simulink model "EPT"  (R2019b)
settings: Solver=FixedStepDiscrete  StartTime=0.0  StopTime=5  FixedStep=0.005  RelTol=1e-3  EnableMultiTasking=on
PreLoadFcn:
  | try, model_open; catch, disp('Error occurred while executing model pre-load callback: model_open.m'); disp('Please assure that the MATLAB working directory is set to the model directory before opening.'); end
InitFcn:
  | try, model_open; catch, end
undefined symbols (not defined in the file or in its folder): Bridge, GCM, H, ln, raptor_get_param_eval, raptor_get_safe_string, raptor_xcp_function
libraries: Raptor_lib x2810, simulink x374, hdlsllib x19
(part 17 of 45)

== system EPT/Foreground_TimeBase_5ms/CAN/CAN2_exec/Remote DA /Remote DA Status G23 (CHGer) ==
  Trigger : TriggerPort  VariantControl=Variant  PortDimensions=1
  raptor_can_txmsg : Raptor_lib/CAN/raptor_can_txmsg  canDefinition=struct('dbcFile', 'EPTvsRemoteDA.dbc','message', 'Remote_DA_Status_G23','comment', '','signals', {{'EPT_OBC_STOP_CTRL','EPT_OBC_IOUT_CMD','EPT_OBC_VOUT_CMD','EPT_OBC_STA','EPT_OBC_CURR','EPT_OBC_VOLT','EPT_OBC_TEMP','EPT_OBC_EW_CODE'}},'enabled', [ 1 1 1 1 1 1 1 1;],'canBus', '''CAN2''','messageID', [ 405008116;],'idMask', [ 536870911;],'payloadMask', [],'payloadValue', [],'period', [ 0;],'mailbox', '','queueSize', [ 1;],'label', [ 1;],'ver', [ 2;],'showID', [ 0;],'showRaw', [ 0;],'fill', [ 0;],'editID', [ 0;],'signalOrder', [ 2;])  canBus='CAN2'  queueSize=1  payloadMask=[]  payloadValue=[]  period=0  showID=0  label=1  idMask=hex2dec('1FFFFFFF')  fill=0  id=405008116  showRaw=0  signalOrder=2  signalInfo={{struct('Name', 'EPT_OBC_VOUT_CMD','Startbit', [ 0;],'SignalSize', [ 8;],'ByteOrder', 'LittleEndian','ValueType', 'UNSIGNED','Class', 'uint8','Signed', [ 0;],'Factor', [ 0.4;],'Offset', [ 0;],'Min', [ 0;],'Max', [ 100;],'Units', '%(Max_Vbatt)','Comment', '','StartBit', [ 16;]),struct('Name', 'EPT_OBC_VOLT','Startbit', [ 0;],'SignalSize', [ 8;],'ByteOrder', 'LittleEndian','ValueType', 'UNSIGNED','Class', 'uint8','Signed', [ 0;],'Factor', [ 0.4;],'Offset', [ 0;],'Min', [ 0;],'Max', [ 100;],'Units', '%(Max_Vchger)','Comment', '','StartBit', [ 40;]),struct('Name', 'EPT_OBC_TEMP','Startbit', [ 0;],'SignalSize', [ 8;],'ByteOrder', 'LittleEndian','ValueType', 'UNSIGNED','Class', 'uint8','Signed', [ 0;],'Factor', [ 1;],'Offset', [ -40;],'Min', [ -40;],'Max', [ 210;],'Units', 'degC','Comment', '','StartBit', [ 48;]),struct('Name', 'EPT_OBC_STOP_CTRL','Startbit', [ 0;],'SignalSize', [ 1;],'ByteOrder', 'LittleEndian','ValueType', 'UNSIGNED','Class', 'uint8','Signed', [ 0;],'Factor', [ 1;],'Offset', [ 0;],'Min', [ 0;],'Max', [ 0;],'Units', '','Comment', '','StartBit', [ 0;]),struct('Name', 'EPT_OBC_STA','Startbit', [ 0;],'SignalSize', [ 1;],'ByteOrder', 'LittleEndian','ValueType', 'UNSIGNED','Class', 'uint8','Signed', [ 0;],'Factor', [ 1;],'Offset', [ 0;],'Min', [ 0;],'Max', [ 0;],'Units', '','Comment', '','StartBit', [ 24;]),struct('Name', 'EPT_OBC_IOUT_CMD','Startbit', [ 0;],'SignalSize', [ 8;],'ByteOrder', 'LittleEndian','ValueType', 'UNSIGNED','Class', 'uint8','Signed', [ 0;],'Factor', [ 0.4;],'Offset', [ 0;],'Min', [ 0;],'Max', [ 100;],'Units', '%(Max Ichger)','Comment', '','StartBit', [ 8;]),struct('Name', 'EPT_OBC_EW_CODE','Startbit', [ 0;],'SignalSize', [ 8;],'ByteOrder', 'LittleEndian','ValueType', 'UNSIGNED','Class', 'uint8','Signed', [ 0;],'Factor', [ 1;],'Offset', [ 0;],'Min', [ 0;],'Max', [ 0;],'Units', '','Comment', '','StartBit', [ 56;]),struct('Name', 'EPT_OBC_CURR','Startbit', [ 0;],'SignalSize', [ 8;],'ByteOrder', 'LittleEndian','ValueType', 'UNSIGNED','Class', 'uint8','Signed', [ 0;],'Factor', [ 0.4;],'Offset', [ 0;],'Min', [ 0;],'Max', [ 100;],'Units', '%(Max Ichger)','Comment', '','StartBit', [ 32;])}}
      settings: SourceProductName=Raptor
  raptor_data_read1 : Raptor_lib/Data Storage/raptor_data_read  dataName='EPT_OBC_VOUT_CMD'  dataShape=Scalar  idxSource=Input  idxRow=1  idxCol=1
      settings: SourceProductName=Raptor
  raptor_data_read2 : Raptor_lib/Data Storage/raptor_data_read  dataName='Read_OBC_Temp'  dataShape=Scalar  idxSource=Input  idxRow=1  idxCol=1
      settings: SourceProductName=Raptor
  raptor_data_read3 : Raptor_lib/Data Storage/raptor_data_read  dataName='EPT_OBC_EN'  dataShape=Scalar  idxSource=Input  idxRow=1  idxCol=1
      settings: SourceProductName=Raptor
  raptor_data_read4 : Raptor_lib/Data Storage/raptor_data_read  dataName='EPT_OBC_STA'  dataShape=Scalar  idxSource=Input  idxRow=1  idxCol=1
      settings: SourceProductName=Raptor
  raptor_data_read5 : Raptor_lib/Data Storage/raptor_data_read  dataName='Read_OBC_Vout'  dataShape=Scalar  idxSource=Input  idxRow=1  idxCol=1
      settings: SourceProductName=Raptor
  raptor_data_read6 : Raptor_lib/Data Storage/raptor_data_read  dataName='Read_OBC_Cout'  dataShape=Scalar  idxSource=Input  idxRow=1  idxCol=1
      settings: SourceProductName=Raptor
  raptor_data_read7 : Raptor_lib/Data Storage/raptor_data_read  dataName='EPT_OBC_IOUT_CMD'  dataShape=Scalar  idxSource=Input  idxRow=1  idxCol=1
      settings: SourceProductName=Raptor
  raptor_data_read8 : Raptor_lib/Data Storage/raptor_data_read  dataName='Read_OBC_Status'  dataShape=Scalar  idxSource=Input  idxRow=1  idxCol=1
      settings: SourceProductName=Raptor
  wires:
  raptor_data_read1/1 -> raptor_can_txmsg/3  "EPT_OBC_VOUT_CMD"
  raptor_data_read3/1 -> raptor_can_txmsg/1  "EPT_OBC_STOP_CTRL"
  raptor_data_read4/1 -> raptor_can_txmsg/4  "EPT_OBC_STA"
  raptor_data_read2/1 -> raptor_can_txmsg/7  "EPT_OBC_TEMP"
  raptor_data_read5/1 -> raptor_can_txmsg/6  "EPT_OBC_VOLT"
  raptor_data_read6/1 -> raptor_can_txmsg/5  "EPT_OBC_CURR"
  raptor_data_read7/1 -> raptor_can_txmsg/2  "EPT_OBC_IOUT_CMD"
  raptor_data_read8/1 -> raptor_can_txmsg/8  "EPT_OBC_EW_CODE"

== system EPT/Foreground_TimeBase_5ms/CAN/CAN2_exec/Remote DA /Remote DA Status G30 (ESS-SWCU) ==
  Trigger : TriggerPort  VariantControl=Variant  PortDimensions=1
  raptor_can_txmsg : Raptor_lib/CAN/raptor_can_txmsg  canDefinition=struct('dbcFile', 'EPTvsRemoteDA.dbc','message', 'Remote_DA_Status_G30','comment', '','signals', {{'EPT_SWCU_READY','EPT_BPSWU_READY','EPT_PWCU_READY','EPT_SWCU_HV_ENABLED','EPT_SWAP_REQ','EPT_BPSWU_INSTALL_NUM','EPT_SWCU_EW_CODE','EPT_BPSWU_FCCAP','EPT_BPSWU_RSOC','EPT_BPSWU_TEMP','EPT_PWCU_CURR_MAX','EPT_PWCU_CURR','EPT_PWCU_TEMP'}},'enabled', [ 1 1 1 1 1 1 1 1 1 1 1 1 1;],'canBus', '''CAN2''','messageID', [ 405860084;],'idMask', [ 536870911;],'payloadMask', [],'payloadValue', [],'period', [ 0;],'mailbox', '','queueSize', [ 1;],'label', [ 0;],'ver', [ 2;],'showID', [ 0;],'showRaw', [ 0;],'fill', [ 0;],'editID', [ 0;],'signalOrder', [ 2;])  canBus='CAN2'  queueSize=1  payloadMask=[]  payloadValue=[]  period=0  showID=0  label=0  idMask=hex2dec('1FFFFFFF')  fill=0  id=405860084  showRaw=0  signalOrder=2  signalInfo={{struct('Name', 'EPT_BPSWU_TEMP','Startbit', [ 0;],'SignalSize', [ 8;],'ByteOrder', 'LittleEndian','ValueType', 'UNSIGNED','Class', 'uint8','Signed', [ 0;],'Factor', [ 1;],'Offset', [ -40;],'Min', [ -40;],'Max', [ 210;],'Units', 'degC','Comment', '','StartBit', [ 32;]),struct('Name', 'EPT_BPSWU_RSOC','Startbit', [ 0;],'SignalSize', [ 8;],'ByteOrder', 'LittleEndian','ValueType', 'UNSIGNED','Class', 'uint8','Signed', [ 0;],'Factor', [ 0.5;],'Offset', [ -12.5;],'Min', [ -12.5;],'Max', [ 112.5;],'Units', 'pct','Comment', '','StartBit', [ 24;]),struct('Name', 'EPT_BPSWU_FCCAP','Startbit', [ 0;],'SignalSize', [ 8;],'ByteOrder', 'LittleEndian','ValueType', 'UNSIGNED','Class', 'uint8','Signed', [ 0;],'Factor', [ 0.4;],'Offset', [ 0;],'Min', [ 0;],'Max', [ 100;],'Units', 'pct (Max_Ah)','Comment', '','StartBit', [ 16;]),struct('Name', 'EPT_SWCU_EW_CODE','Startbit', [ 0;],'SignalSize', [ 8;],'ByteOrder', 'LittleEndian','ValueType', 'UNSIGNED','Class', 'uint8','Signed', [ 0;],'Factor', [ 1;],'Offset', [ 0;],'Min', [ 0;],'Max', [ 0;],'Units', '','Comment', '','StartBit', [ 8;]),struct('Name', 'EPT_PWCU_TEMP','Startbit', [ 0;],'SignalSize', [ 8;],'ByteOrder', 'LittleEndian','ValueType', 'UNSIGNED','Class', 'uint8','Signed', [ 0;],'Factor', [ 1;],'Offset', [ -40;],'Min', [ -40;],'Max', [ 210;],'Units', 'degC','Comment', '','StartBit', [ 56;]),struct('Name', 'EPT_PWCU_CURR_MAX','Startbit', [ 0;],'SignalSize', [ 8;],'ByteOrder', 'LittleEndian','ValueType', 'UNSIGNED','Class', 'uint8','Signed', [ 0;],'Factor', [ 0.4;],'Offset', [ 0;],'Min', [ 0;],'Max', [ 100;],'Units', '% (Imax)','Comment', '','StartBit', [ 40;]),struct('Name', 'EPT_PWCU_CURR','Startbit', [ 0;],'SignalSize', [ 8;],'ByteOrder', 'LittleEndian','ValueType', 'UNSIGNED','Class', 'uint8','Signed', [ 0;],'Factor', [ 0.4;],'Offset', [ 0;],'Min', [ 0;],'Max', [ 100;],'Units', '% (Imax)','Comment', '','StartBit', [ 48;]),struct('Name', 'EPT_BPSWU_INSTALL_NUM','Startbit', [ 0;],'SignalSize', [ 3;],'ByteOrder', 'LittleEndian','ValueType', 'UNSIGNED','Class', 'uint8','Signed', [ 0;],'Factor', [ 1;],'Offset', [ 0;],'Min', [ 0;],'Max', [ 0;],'Units', '','Comment', '','StartBit', [ 5;]),struct('Name', 'EPT_SWCU_READY','Startbit', [ 0;],'SignalSize', [ 1;],'ByteOrder', 'LittleEndian','ValueType', 'UNSIGNED','Class', 'uint8','Signed', [ 0;],'Factor', [ 1;],'Offset', [ 0;],'Min', [ 0;],'Max', [ 0;],'Units', '','Comment', '','StartBit', [ 0;]),struct('Name', 'EPT_SWCU_HV_ENABLED','Startbit', [ 0;],'SignalSize', [ 1;],'ByteOrder', 'LittleEndian','ValueType', 'UNSIGNED','Class', 'uint8','Signed', [ 0;],'Factor', [ 1;],'Offset', [ 0;],'Min', [ 0;],'Max', [ 0;],'Units', '','Comment', '','StartBit', [ 3;]),struct('Name', 'EPT_SWAP_REQ','Startbit', [ 0;],'SignalSize', [ 1;],'ByteOrder', 'LittleEndian','ValueType', 'UNSIGNED','Class', 'uint8','Signed', [ 0;],'Factor', [ 1;],'Offset', [ 0;],'Min', [ 0;],'Max', [ 0;],'Units', '','Comment', '','StartBit', [ 4;]),struct('Name', 'EPT_PWCU_READY','Startbit', [ 0;],'SignalSize', [ 1;],'ByteOrder', 'LittleEndian','ValueType', 'UNSIGNED','Class', 'uint8','Signed', [ 0;],'Factor', [ 1;],'Offset', [ 0;],'Min', [ 0;],'Max', [ 0;],'Units', '','Comment', '','StartBit', [ 2;]),struct('Name', 'EPT_BPSWU_READY','Startbit', [ 0;],'SignalSize', [ 1;],'ByteOrder', 'LittleEndian','ValueType', 'UNSIGNED','Class', 'uint8','Signed', [ 0;],'Factor', [ 1;],'Offset', [ 0;],'Min', [ 0;],'Max', [ 0;],'Units', '','Comment', '','StartBit', [ 1;])}}
      settings: SourceProductName=Raptor
  raptor_data_read : Raptor_lib/Data Storage/raptor_data_read  dataName='SWCU_PWCU_READY'  dataShape=Scalar  idxSource=Input  idxRow=1  idxCol=1
      settings: SourceProductName=Raptor
  raptor_data_read1 : Raptor_lib/Data Storage/raptor_data_read  dataName='SWCU_HV_ENABLED'  dataShape=Scalar  idxSource=Input  idxRow=1  idxCol=1
      settings: SourceProductName=Raptor
  raptor_data_read10 : Raptor_lib/Data Storage/raptor_data_read  dataName='SWCU_BPSWU_FCCAP'  dataShape=Scalar  idxSource=Input  idxRow=1  idxCol=1
      settings: SourceProductName=Raptor
  raptor_data_read11 : Raptor_lib/Data Storage/raptor_data_read  dataName='SWCU_PWCU_IOUT'  dataShape=Scalar  idxSource=Input  idxRow=1  idxCol=1
      settings: SourceProductName=Raptor
  raptor_data_read2 : Raptor_lib/Data Storage/raptor_data_read  dataName='SWCU_SWAP_REQUEST'  dataShape=Scalar  idxSource=Input  idxRow=1  idxCol=1
      settings: SourceProductName=Raptor
  raptor_data_read3 : Raptor_lib/Data Storage/raptor_data_read  dataName='SWCU_BPSWU_INSTALL_NUM'  dataShape=Scalar  idxSource=Input  idxRow=1  idxCol=1
      settings: SourceProductName=Raptor
  raptor_data_read4 : Raptor_lib/Data Storage/raptor_data_read  dataName='SWCU_EW_CODE'  dataShape=Scalar  idxSource=Input  idxRow=1  idxCol=1
      settings: SourceProductName=Raptor
  raptor_data_read5 : Raptor_lib/Data Storage/raptor_data_read  dataName='SWCU_BPSWU_TEMP'  dataShape=Scalar  idxSource=Input  idxRow=1  idxCol=1
      settings: SourceProductName=Raptor
  raptor_data_read6 : Raptor_lib/Data Storage/raptor_data_read  dataName='SWCU_PWCU_TEMP'  dataShape=Scalar  idxSource=Input  idxRow=1  idxCol=1
      settings: SourceProductName=Raptor
  raptor_data_read7 : Raptor_lib/Data Storage/raptor_data_read  dataName='SWCU_BPSWU_READY'  dataShape=Scalar  idxSource=Input  idxRow=1  idxCol=1
      settings: SourceProductName=Raptor
  raptor_data_read8 : Raptor_lib/Data Storage/raptor_data_read  dataName='SWCU_READY'  dataShape=Scalar  idxSource=Input  idxRow=1  idxCol=1
      settings: SourceProductName=Raptor
  raptor_data_read9 : Raptor_lib/Data Storage/raptor_data_read  dataName='SWCU_BPSWU_RSOC'  dataShape=Scalar  idxSource=Input  idxRow=1  idxCol=1
      settings: SourceProductName=Raptor
  wires:
  raptor_data_read/1 -> raptor_can_txmsg/3
  raptor_data_read1/1 -> raptor_can_txmsg/4
  raptor_data_read2/1 -> raptor_can_txmsg/5
  raptor_data_read7/1 -> raptor_can_txmsg/2
  raptor_data_read8/1 -> raptor_can_txmsg/1
  raptor_data_read9/1 -> raptor_can_txmsg/9
  raptor_data_read10/1 -> raptor_can_txmsg/8
  raptor_data_read3/1 -> raptor_can_txmsg/6
  raptor_data_read4/1 -> raptor_can_txmsg/7
  raptor_data_read5/1 -> raptor_can_txmsg/10
  raptor_data_read6/1 -> raptor_can_txmsg/13
  raptor_data_read11/1 -> raptor_can_txmsg/12

== system EPT/Foreground_TimeBase_5ms/CAN/CAN2_exec/Remote DA /Remote DA Status G31 (ESS-SWUBP#1) ==
  Trigger : TriggerPort  VariantControl=Variant  PortDimensions=1
  raptor_can_txmsg : Raptor_lib/CAN/raptor_can_txmsg  canDefinition=struct('dbcFile', 'EPTvsRemoteDA.dbc','message', 'Remote_DA_Status_G31','comment', '','signals', {{'EPT_BPSWU1_READY','EPT_BPSWU1_HV_ENABLED','EPT_BPSWU1_EW','EPT_BPSWU1_EW_CODE','EPT_BPSWU1_FCCAP','EPT_BPSWU1_RSOC','EPT_BPSWU1_CURR','EPT_BPSWU1_VOLT','EPT_BPSWU1_TEMP','EPT_BPSWU1_VCELL_MAX','EPT_BPSWU1_VCELL_MIN'}},'enabled', [ 1 1 1 1 1 1 1 1 1 1 1;],'canBus', '''CAN2''','messageID', [ 405925620;],'idMask', [ 536870911;],'payloadMask', [],'payloadValue', [],'period', [ 0;],'mailbox', '','queueSize', [ 1;],'label', [ 0;],'ver', [ 2;],'showID', [ 0;],'showRaw', [ 0;],'fill', [ 0;],'editID', [ 0;],'signalOrder', [ 2;])  canBus='CAN2'  queueSize=1  payloadMask=[]  payloadValue=[]  period=0  showID=0  label=0  idMask=hex2dec('1FFFFFFF')  fill=0  id=405925620  showRaw=0  signalOrder=2  signalInfo={{struct('Name', 'EPT_BPSWU1_VOLT','Startbit', [ 0;],'SignalSize', [ 8;],'ByteOrder', 'LittleEndian','ValueType', 'UNSIGNED','Class', 'uint8','Signed', [ 0;],'Factor', [ 0.4;],'Offset', [ 0;],'Min', [ 0;],'Max', [ 100;],'Units', 'pct (Max_Vbatt)','Comment', '','StartBit', [ 32;]),struct('Name', 'EPT_BPSWU1_VCELL_MIN','Startbit', [ 0;],'SignalSize', [ 8;],'ByteOrder', 'LittleEndian','ValueType', 'UNSIGNED','Class', 'uint8','Signed', [ 0;],'Factor', [ 0.01;],'Offset', [ 2;],'Min', [ 2;],'Max', [ 4.5;],'Units', 'Volt','Comment', '','StartBit', [ 56;]),struct('Name', 'EPT_BPSWU1_VCELL_MAX','Startbit', [ 0;],'SignalSize', [ 8;],'ByteOrder', 'LittleEndian','ValueType', 'UNSIGNED','Class', 'uint8','Signed', [ 0;],'Factor', [ 0.01;],'Offset', [ 2;],'Min', [ 2;],'Max', [ 4.5;],'Units', 'Volt','Comment', '','StartBit', [ 48;]),struct('Name', 'EPT_BPSWU1_TEMP','Startbit', [ 0;],'SignalSize', [ 8;],'ByteOrder', 'LittleEndian','ValueType', 'UNSIGNED','Class', 'uint8','Signed', [ 0;],'Factor', [ 1;],'Offset', [ -40;],'Min', [ -40;],'Max', [ 210;],'Units', 'degC','Comment', '','StartBit', [ 40;]),struct('Name', 'EPT_BPSWU1_RSOC','Startbit', [ 0;],'SignalSize', [ 8;],'ByteOrder', 'LittleEndian','ValueType', 'UNSIGNED','Class', 'uint8','Signed', [ 0;],'Factor', [ 1;],'Offset', [ 0;],'Min', [ 0;],'Max', [ 0;],'Units', '','Comment', '','StartBit', [ 16;]),struct('Name', 'EPT_BPSWU1_FCCAP','Startbit', [ 0;],'SignalSize', [ 8;],'ByteOrder', 'LittleEndian','ValueType', 'UNSIGNED','Class', 'uint8','Signed', [ 0;],'Factor', [ 0.4;],'Offset', [ 0;],'Min', [ 0;],'Max', [ 100;],'Units', 'pct (Max_Ah)','Comment', '','StartBit', [ 8;]),struct('Name', 'EPT_BPSWU1_CURR','Startbit', [ 0;],'SignalSize', [ 8;],'ByteOrder', 'LittleEndian','ValueType', 'UNSIGNED','Class', 'uint8','Signed', [ 0;],'Factor', [ 0.8;],'Offset', [ -100;],'Min', [ -100;],'Max', [ 100;],'Units', 'pct (Max Ibatt)','Comment', '','StartBit', [ 24;]),struct('Name', 'EPT_BPSWU1_EW_CODE','Startbit', [ 0;],'SignalSize', [ 5;],'ByteOrder', 'LittleEndian','ValueType', 'UNSIGNED','Class', 'uint8','Signed', [ 0;],'Factor', [ 1;],'Offset', [ 0;],'Min', [ 0;],'Max', [ 0;],'Units', '','Comment', '','StartBit', [ 3;]),struct('Name', 'EPT_BPSWU1_READY','Startbit', [ 0;],'SignalSize', [ 1;],'ByteOrder', 'LittleEndian','ValueType', 'UNSIGNED','Class', 'uint8','Signed', [ 0;],'Factor', [ 1;],'Offset', [ 0;],'Min', [ 0;],'Max', [ 0;],'Units', '','Comment', '','StartBit', [ 0;]),struct('Name', 'EPT_BPSWU1_HV_ENABLED','Startbit', [ 0;],'SignalSize', [ 1;],'ByteOrder', 'LittleEndian','ValueType', 'UNSIGNED','Class', 'uint8','Signed', [ 0;],'Factor', [ 1;],'Offset', [ 0;],'Min', [ 0;],'Max', [ 0;],'Units', '','Comment', '','StartBit', [ 1;]),struct('Name', 'EPT_BPSWU1_EW','Startbit', [ 0;],'SignalSize', [ 1;],'ByteOrder', 'LittleEndian','ValueType', 'UNSIGNED','Class', 'uint8','Signed', [ 0;],'Factor', [ 1;],'Offset', [ 0;],'Min', [ 0;],'Max', [ 0;],'Units', '','Comment', '','StartBit', [ 2;])}}
      settings: SourceProductName=Raptor
  raptor_data_read : Raptor_lib/Data Storage/raptor_data_read  dataName='SWCU_BPSWU1_READY'  dataShape=Scalar  idxSource=Input  idxRow=1  idxCol=1
      settings: SourceProductName=Raptor
  raptor_data_read1 : Raptor_lib/Data Storage/raptor_data_read  dataName='SWCU_BPSWU1_HV_ENABLED'  dataShape=Scalar  idxSource=Input  idxRow=1  idxCol=1
      settings: SourceProductName=Raptor
  raptor_data_read10 : Raptor_lib/Data Storage/raptor_data_read  dataName='SWCU_BPSWU1_VCELL_MIN'  dataShape=Scalar  idxSource=Input  idxRow=1  idxCol=1
      settings: SourceProductName=Raptor
  raptor_data_read2 : Raptor_lib/Data Storage/raptor_data_read  dataName='SWCU_BPSWU1_EW'  dataShape=Scalar  idxSource=Input  idxRow=1  idxCol=1
      settings: SourceProductName=Raptor
  raptor_data_read3 : Raptor_lib/Data Storage/raptor_data_read  dataName='SWCU_BPSWU1_EW_CODE'  dataShape=Scalar  idxSource=Input  idxRow=1  idxCol=1
      settings: SourceProductName=Raptor
  raptor_data_read4 : Raptor_lib/Data Storage/raptor_data_read  dataName='SWCU_BPSWU1_FCCAP'  dataShape=Scalar  idxSource=Input  idxRow=1  idxCol=1
      settings: SourceProductName=Raptor
  raptor_data_read5 : Raptor_lib/Data Storage/raptor_data_read  dataName='SWCU_BPSWU1_RSOC'  dataShape=Scalar  idxSource=Input  idxRow=1  idxCol=1
      settings: SourceProductName=Raptor
  raptor_data_read6 : Raptor_lib/Data Storage/raptor_data_read  dataName='SWCU_BPSWU1_CURR'  dataShape=Scalar  idxSource=Input  idxRow=1  idxCol=1
      settings: SourceProductName=Raptor
  raptor_data_read7 : Raptor_lib/Data Storage/raptor_data_read  dataName='SWCU_BPSWU1_VOLT'  dataShape=Scalar  idxSource=Input  idxRow=1  idxCol=1
      settings: SourceProductName=Raptor
  raptor_data_read8 : Raptor_lib/Data Storage/raptor_data_read  dataName='SWCU_BPSWU1_TEMP'  dataShape=Scalar  idxSource=Input  idxRow=1  idxCol=1
      settings: SourceProductName=Raptor
  raptor_data_read9 : Raptor_lib/Data Storage/raptor_data_read  dataName='SWCU_BPSWU1_VCELL_MAX'  dataShape=Scalar  idxSource=Input  idxRow=1  idxCol=1
      settings: SourceProductName=Raptor
  wires:
  raptor_data_read/1 -> raptor_can_txmsg/1
  raptor_data_read1/1 -> raptor_can_txmsg/2
  raptor_data_read3/1 -> raptor_can_txmsg/4
  raptor_data_read2/1 -> raptor_can_txmsg/3
  raptor_data_read6/1 -> raptor_can_txmsg/7
  raptor_data_read7/1 -> raptor_can_txmsg/8
  raptor_data_read5/1 -> raptor_can_txmsg/6
  raptor_data_read4/1 -> raptor_can_txmsg/5
  raptor_data_read8/1 -> raptor_can_txmsg/9
  raptor_data_read9/1 -> raptor_can_txmsg/10
  raptor_data_read10/1 -> raptor_can_txmsg/11

== system EPT/Foreground_TimeBase_5ms/CAN/CAN2_exec/Remote DA /Remote DA Status G32 (ESS-SWUBP#2) ==
  Trigger : TriggerPort  VariantControl=Variant  PortDimensions=1
  raptor_can_txmsg : Raptor_lib/CAN/raptor_can_txmsg  canDefinition=struct('dbcFile', 'EPTvsRemoteDA.dbc','message', 'Remote_DA_Status_G32','comment', '','signals', {{'EPT_BPSWU2_CURR','EPT_BPSWU2_EW','EPT_BPSWU2_EW_CODE','EPT_BPSWU2_FCCAP','EPT_BPSWU2_HV_ENABLED','EPT_BPSWU2_READY','EPT_BPSWU2_RSOC','EPT_BPSWU2_TEMP','EPT_BPSWU2_VCELL_MAX','EPT_BPSWU2_VCELL_MIN','EPT_BPSWU2_VOLT'}},'enabled', [ 1 1 1 1 1 1 1 1 1 1 1;],'canBus', '''CAN2''','messageID', [ 405991156;],'idMask', [ 536870911;],'payloadMask', [],'payloadValue', [],'period', [ 0;],'mailbox', '','queueSize', [ 1;],'label', [ 0;],'ver', [ 2;],'showID', [ 0;],'showRaw', [ 0;],'fill', [ 0;],'editID', [ 0;],'signalOrder', [ 1;])  canBus='CAN2'  queueSize=1  payloadMask=[]  payloadValue=[]  period=0  showID=0  label=0  idMask=hex2dec('1FFFFFFF')  fill=0  id=405991156  showRaw=0  signalOrder=1  signalInfo={{struct('Name', 'EPT_BPSWU2_VOLT','Startbit', [ 0;],'SignalSize', [ 8;],'ByteOrder', 'LittleEndian','ValueType', 'UNSIGNED','Class', 'uint8','Signed', [ 0;],'Factor', [ 0.4;],'Offset', [ 0;],'Min', [ 0;],'Max', [ 100;],'Units', 'pct (Max_Vbatt)','Comment', '','StartBit', [ 32;]),struct('Name', 'EPT_BPSWU2_VCELL_MIN','Startbit', [ 0;],'SignalSize', [ 8;],'ByteOrder', 'LittleEndian','ValueType', 'UNSIGNED','Class', 'uint8','Signed', [ 0;],'Factor', [ 0.01;],'Offset', [ 2;],'Min', [ 2;],'Max', [ 4.5;],'Units', 'Volt','Comment', '','StartBit', [ 56;]),struct('Name', 'EPT_BPSWU2_VCELL_MAX','Startbit', [ 0;],'SignalSize', [ 8;],'ByteOrder', 'LittleEndian','ValueType', 'UNSIGNED','Class', 'uint8','Signed', [ 0;],'Factor', [ 0.01;],'Offset', [ 2;],'Min', [ 2;],'Max', [ 4.5;],'Units', 'Volt','Comment', '','StartBit', [ 48;]),struct('Name', 'EPT_BPSWU2_TEMP','Startbit', [ 0;],'SignalSize', [ 8;],'ByteOrder', 'LittleEndian','ValueType', 'UNSIGNED','Class', 'uint8','Signed', [ 0;],'Factor', [ 1;],'Offset', [ -40;],'Min', [ -40;],'Max', [ 210;],'Units', 'degC','Comment', '','StartBit', [ 40;]),struct('Name', 'EPT_BPSWU2_RSOC','Startbit', [ 0;],'SignalSize', [ 8;],'ByteOrder', 'LittleEndian','ValueType', 'UNSIGNED','Class', 'uint8','Signed', [ 0;],'Factor', [ 1;],'Offset', [ 0;],'Min', [ 0;],'Max', [ 0;],'Units', '','Comment', '','StartBit', [ 16;]),struct('Name', 'EPT_BPSWU2_READY','Startbit', [ 0;],'SignalSize', [ 1;],'ByteOrder', 'LittleEndian','ValueType', 'UNSIGNED','Class', 'uint8','Signed', [ 0;],'Factor', [ 1;],'Offset', [ 0;],'Min', [ 0;],'Max', [ 0;],'Units', '','Comment', '','StartBit', [ 0;]),struct('Name', 'EPT_BPSWU2_HV_ENABLED','Startbit', [ 0;],'SignalSize', [ 1;],'ByteOrder', 'LittleEndian','ValueType', 'UNSIGNED','Class', 'uint8','Signed', [ 0;],'Factor', [ 1;],'Offset', [ 0;],'Min', [ 0;],'Max', [ 0;],'Units', '','Comment', '','StartBit', [ 1;]),struct('Name', 'EPT_BPSWU2_FCCAP','Startbit', [ 0;],'SignalSize', [ 8;],'ByteOrder', 'LittleEndian','ValueType', 'UNSIGNED','Class', 'uint8','Signed', [ 0;],'Factor', [ 0.4;],'Offset', [ 0;],'Min', [ 0;],'Max', [ 100;],'Units', 'pct (Max_Ah)','Comment', '','StartBit', [ 8;]),struct('Name', 'EPT_BPSWU2_EW_CODE','Startbit', [ 0;],'SignalSize', [ 5;],'ByteOrder', 'LittleEndian','ValueType', 'UNSIGNED','Class', 'uint8','Signed', [ 0;],'Factor', [ 1;],'Offset', [ 0;],'Min', [ 0;],'Max', [ 0;],'Units', '','Comment', '','StartBit', [ 3;]),struct('Name', 'EPT_BPSWU2_EW','Startbit', [ 0;],'SignalSize', [ 1;],'ByteOrder', 'LittleEndian','ValueType', 'UNSIGNED','Class', 'uint8','Signed', [ 0;],'Factor', [ 1;],'Offset', [ 0;],'Min', [ 0;],'Max', [ 0;],'Units', '','Comment', '','StartBit', [ 2;]),struct('Name', 'EPT_BPSWU2_CURR','Startbit', [ 0;],'SignalSize', [ 8;],'ByteOrder', 'LittleEndian','ValueType', 'UNSIGNED','Class', 'uint8','Signed', [ 0;],'Factor', [ 0.8;],'Offset', [ -100;],'Min', [ -100;],'Max', [ 100;],'Units', 'pct (Max Ibatt)','Comment', '','StartBit', [ 24;])}}
      settings: SourceProductName=Raptor
  raptor_data_read : Raptor_lib/Data Storage/raptor_data_read  dataName='SWCU_BPSWU2_READY'  dataShape=Scalar  idxSource=Input  idxRow=1  idxCol=1
      settings: SourceProductName=Raptor
  raptor_data_read1 : Raptor_lib/Data Storage/raptor_data_read  dataName='SWCU_BPSWU2_HV_ENABLED'  dataShape=Scalar  idxSource=Input  idxRow=1  idxCol=1
      settings: SourceProductName=Raptor
  raptor_data_read10 : Raptor_lib/Data Storage/raptor_data_read  dataName='SWCU_BPSWU2_VCELL_MIN'  dataShape=Scalar  idxSource=Input  idxRow=1  idxCol=1
      settings: SourceProductName=Raptor
  raptor_data_read2 : Raptor_lib/Data Storage/raptor_data_read  dataName='SWCU_BPSWU2_EW'  dataShape=Scalar  idxSource=Input  idxRow=1  idxCol=1
      settings: SourceProductName=Raptor
  raptor_data_read3 : Raptor_lib/Data Storage/raptor_data_read  dataName='SWCU_BPSWU2_EW_CODE'  dataShape=Scalar  idxSource=Input  idxRow=1  idxCol=1
      settings: SourceProductName=Raptor
  raptor_data_read4 : Raptor_lib/Data Storage/raptor_data_read  dataName='SWCU_BPSWU2_FCCAP'  dataShape=Scalar  idxSource=Input  idxRow=1  idxCol=1
      settings: SourceProductName=Raptor
  raptor_data_read5 : Raptor_lib/Data Storage/raptor_data_read  dataName='SWCU_BPSWU2_RSOC'  dataShape=Scalar  idxSource=Input  idxRow=1  idxCol=1
      settings: SourceProductName=Raptor
  raptor_data_read6 : Raptor_lib/Data Storage/raptor_data_read  dataName='SWCU_BPSWU2_CURR'  dataShape=Scalar  idxSource=Input  idxRow=1  idxCol=1
      settings: SourceProductName=Raptor
  raptor_data_read7 : Raptor_lib/Data Storage/raptor_data_read  dataName='SWCU_BPSWU2_VOLT'  dataShape=Scalar  idxSource=Input  idxRow=1  idxCol=1
      settings: SourceProductName=Raptor
  raptor_data_read8 : Raptor_lib/Data Storage/raptor_data_read  dataName='SWCU_BPSWU2_TEMP'  dataShape=Scalar  idxSource=Input  idxRow=1  idxCol=1
      settings: SourceProductName=Raptor
  raptor_data_read9 : Raptor_lib/Data Storage/raptor_data_read  dataName='SWCU_BPSWU2_VCELL_MAX'  dataShape=Scalar  idxSource=Input  idxRow=1  idxCol=1
      settings: SourceProductName=Raptor
  wires:
  raptor_data_read1/1 -> raptor_can_txmsg/2
  raptor_data_read9/1 -> raptor_can_txmsg/10
  raptor_data_read6/1 -> raptor_can_txmsg/7
  raptor_data_read7/1 -> raptor_can_txmsg/8
  raptor_data_read3/1 -> raptor_can_txmsg/4
  raptor_data_read4/1 -> raptor_can_txmsg/5
  raptor_data_read8/1 -> raptor_can_txmsg/9
  raptor_data_read10/1 -> raptor_can_txmsg/11
  raptor_data_read/1 -> raptor_can_txmsg/1
  raptor_data_read5/1 -> raptor_can_txmsg/6
  raptor_data_read2/1 -> raptor_can_txmsg/3

== system EPT/Foreground_TimeBase_5ms/CAN/CAN2_exec/Remote DA /Remote DA Status G33 (ESS-SWUBP#3) ==
  Trigger : TriggerPort  VariantControl=Variant  PortDimensions=1
  raptor_can_txmsg : Raptor_lib/CAN/raptor_can_txmsg  canDefinition=struct('dbcFile', 'EPTvsRemoteDA.dbc','message', 'Remote_DA_Status_G33','comment', '','signals', {{'EPT_BPSWU3_CURR','EPT_BPSWU3_EW','EPT_BPSWU3_EW_CODE','EPT_BPSWU3_FCCAP','EPT_BPSWU3_HV_ENABLED','EPT_BPSWU3_READY','EPT_BPSWU3_RSOC','EPT_BPSWU3_TEMP','EPT_BPSWU3_VCELL_MAX','EPT_BPSWU3_VCELL_MIN','EPT_BPSWU3_VOLT'}},'enabled', [ 1 1 1 1 1 1 1 1 1 1 1;],'canBus', '''CAN2''','messageID', [ 406056692;],'idMask', [ 536870911;],'payloadMask', [],'payloadValue', [],'period', [ 0;],'mailbox', '','queueSize', [ 1;],'label', [ 0;],'ver', [ 2;],'showID', [ 0;],'showRaw', [ 0;],'fill', [ 0;],'editID', [ 0;],'signalOrder', [ 1;])  canBus='CAN2'  queueSize=1  payloadMask=[]  payloadValue=[]  period=0  showID=0  label=0  idMask=hex2dec('1FFFFFFF')  fill=0  id=406056692  showRaw=0  signalOrder=1  signalInfo={{struct('Name', 'EPT_BPSWU3_VOLT','Startbit', [ 0;],'SignalSize', [ 8;],'ByteOrder', 'LittleEndian','ValueType', 'UNSIGNED','Class', 'uint8','Signed', [ 0;],'Factor', [ 0.4;],'Offset', [ 0;],'Min', [ 0;],'Max', [ 100;],'Units', 'pct (Max_Vbatt)','Comment', '','StartBit', [ 32;]),struct('Name', 'EPT_BPSWU3_VCELL_MIN','Startbit', [ 0;],'SignalSize', [ 8;],'ByteOrder', 'LittleEndian','ValueType', 'UNSIGNED','Class', 'uint8','Signed', [ 0;],'Factor', [ 0.01;],'Offset', [ 2;],'Min', [ 2;],'Max', [ 4.5;],'Units', 'Volt','Comment', '','StartBit', [ 56;]),struct('Name', 'EPT_BPSWU3_VCELL_MAX','Startbit', [ 0;],'SignalSize', [ 8;],'ByteOrder', 'LittleEndian','ValueType', 'UNSIGNED','Class', 'uint8','Signed', [ 0;],'Factor', [ 0.01;],'Offset', [ 2;],'Min', [ 2;],'Max', [ 4.5;],'Units', 'Volt','Comment', '','StartBit', [ 48;]),struct('Name', 'EPT_BPSWU3_TEMP','Startbit', [ 0;],'SignalSize', [ 8;],'ByteOrder', 'LittleEndian','ValueType', 'UNSIGNED','Class', 'uint8','Signed', [ 0;],'Factor', [ 1;],'Offset', [ -40;],'Min', [ -40;],'Max', [ 210;],'Units', 'degC','Comment', '','StartBit', [ 40;]),struct('Name', 'EPT_BPSWU3_RSOC','Startbit', [ 0;],'SignalSize', [ 8;],'ByteOrder', 'LittleEndian','ValueType', 'UNSIGNED','Class', 'uint8','Signed', [ 0;],'Factor', [ 1;],'Offset', [ 0;],'Min', [ 0;],'Max', [ 0;],'Units', '','Comment', '','StartBit', [ 16;]),struct('Name', 'EPT_BPSWU3_READY','Startbit', [ 0;],'SignalSize', [ 1;],'ByteOrder', 'LittleEndian','ValueType', 'UNSIGNED','Class', 'uint8','Signed', [ 0;],'Factor', [ 1;],'Offset', [ 0;],'Min', [ 0;],'Max', [ 0;],'Units', '','Comment', '','StartBit', [ 0;]),struct('Name', 'EPT_BPSWU3_HV_ENABLED','Startbit', [ 0;],'SignalSize', [ 1;],'ByteOrder', 'LittleEndian','ValueType', 'UNSIGNED','Class', 'uint8','Signed', [ 0;],'Factor', [ 1;],'Offset', [ 0;],'Min', [ 0;],'Max', [ 0;],'Units', '','Comment', '','StartBit', [ 1;]),struct('Name', 'EPT_BPSWU3_FCCAP','Startbit', [ 0;],'SignalSize', [ 8;],'ByteOrder', 'LittleEndian','ValueType', 'UNSIGNED','Class', 'uint8','Signed', [ 0;],'Factor', [ 0.4;],'Offset', [ 0;],'Min', [ 0;],'Max', [ 100;],'Units', 'pct (Max_Ah)','Comment', '','StartBit', [ 8;]),struct('Name', 'EPT_BPSWU3_EW_CODE','Startbit', [ 0;],'SignalSize', [ 5;],'ByteOrder', 'LittleEndian','ValueType', 'UNSIGNED','Class', 'uint8','Signed', [ 0;],'Factor', [ 1;],'Offset', [ 0;],'Min', [ 0;],'Max', [ 0;],'Units', '','Comment', '','StartBit', [ 3;]),struct('Name', 'EPT_BPSWU3_EW','Startbit', [ 0;],'SignalSize', [ 1;],'ByteOrder', 'LittleEndian','ValueType', 'UNSIGNED','Class', 'uint8','Signed', [ 0;],'Factor', [ 1;],'Offset', [ 0;],'Min', [ 0;],'Max', [ 0;],'Units', '','Comment', '','StartBit', [ 2;]),struct('Name', 'EPT_BPSWU3_CURR','Startbit', [ 0;],'SignalSize', [ 8;],'ByteOrder', 'LittleEndian','ValueType', 'UNSIGNED','Class', 'uint8','Signed', [ 0;],'Factor', [ 0.8;],'Offset', [ -100;],'Min', [ -100;],'Max', [ 100;],'Units', 'pct (Max Ibatt)','Comment', '','StartBit', [ 24;])}}
      settings: SourceProductName=Raptor
  raptor_data_read : Raptor_lib/Data Storage/raptor_data_read  dataName='SWCU_BPSWU3_READY'  dataShape=Scalar  idxSource=Input  idxRow=1  idxCol=1
      settings: SourceProductName=Raptor
  raptor_data_read1 : Raptor_lib/Data Storage/raptor_data_read  dataName='SWCU_BPSWU3_HV_ENABLED'  dataShape=Scalar  idxSource=Input  idxRow=1  idxCol=1
      settings: SourceProductName=Raptor
  raptor_data_read10 : Raptor_lib/Data Storage/raptor_data_read  dataName='SWCU_BPSWU3_VCELL_MIN'  dataShape=Scalar  idxSource=Input  idxRow=1  idxCol=1
      settings: SourceProductName=Raptor
  raptor_data_read2 : Raptor_lib/Data Storage/raptor_data_read  dataName='SWCU_BPSWU3_EW'  dataShape=Scalar  idxSource=Input  idxRow=1  idxCol=1
      settings: SourceProductName=Raptor
  raptor_data_read3 : Raptor_lib/Data Storage/raptor_data_read  dataName='SWCU_BPSWU3_EW_CODE'  dataShape=Scalar  idxSource=Input  idxRow=1  idxCol=1
      settings: SourceProductName=Raptor
  raptor_data_read4 : Raptor_lib/Data Storage/raptor_data_read  dataName='SWCU_BPSWU3_FCCAP'  dataShape=Scalar  idxSource=Input  idxRow=1  idxCol=1
      settings: SourceProductName=Raptor
  raptor_data_read5 : Raptor_lib/Data Storage/raptor_data_read  dataName='SWCU_BPSWU3_RSOC'  dataShape=Scalar  idxSource=Input  idxRow=1  idxCol=1
      settings: SourceProductName=Raptor
  raptor_data_read6 : Raptor_lib/Data Storage/raptor_data_read  dataName='SWCU_BPSWU3_CURR'  dataShape=Scalar  idxSource=Input  idxRow=1  idxCol=1
      settings: SourceProductName=Raptor
  raptor_data_read7 : Raptor_lib/Data Storage/raptor_data_read  dataName='SWCU_BPSWU3_VOLT'  dataShape=Scalar  idxSource=Input  idxRow=1  idxCol=1
      settings: SourceProductName=Raptor
  raptor_data_read8 : Raptor_lib/Data Storage/raptor_data_read  dataName='SWCU_BPSWU3_TEMP'  dataShape=Scalar  idxSource=Input  idxRow=1  idxCol=1
      settings: SourceProductName=Raptor
  raptor_data_read9 : Raptor_lib/Data Storage/raptor_data_read  dataName='SWCU_BPSWU3_VCELL_MAX'  dataShape=Scalar  idxSource=Input  idxRow=1  idxCol=1
      settings: SourceProductName=Raptor
  wires:
  raptor_data_read10/1 -> raptor_can_txmsg/11
  raptor_data_read6/1 -> raptor_can_txmsg/7
  raptor_data_read/1 -> raptor_can_txmsg/1
  raptor_data_read7/1 -> raptor_can_txmsg/8
  raptor_data_read4/1 -> raptor_can_txmsg/5
  raptor_data_read5/1 -> raptor_can_txmsg/6
  raptor_data_read2/1 -> raptor_can_txmsg/3
  raptor_data_read8/1 -> raptor_can_txmsg/9
  raptor_data_read9/1 -> raptor_can_txmsg/10
  raptor_data_read1/1 -> raptor_can_txmsg/2
  raptor_data_read3/1 -> raptor_can_txmsg/4

== system EPT/Foreground_TimeBase_5ms/CAN/CAN3_exec/20CH_TCS/CH13_CH16_Rx ==
  Factor : Inport
  Offset : Inport  Port=2
  Trigger : TriggerPort  VariantControl=Variant  PortDimensions=1
  Convert_Byte2Data : Subsystem
  Convert_Byte2Data1 : Subsystem
  Convert_Byte2Data2 : Subsystem
  Convert_Byte2Data3 : Subsystem
  Demux : Demux  Outputs=8
  raptor_can_rxraw : Raptor_lib/CAN/raptor_can_rxraw  canBus='CAN3'  extendedId=1  showAge=1  id=hex2dec('18FEA0EB')  idMask=hex2dec('1FFFFFFF')  mailbox=''  queueSize=1
      settings: SourceProductName=Raptor
  raptor_measurement : Raptor_lib/Data Storage/raptor_measurement  paramName='T13'  nameSource=Parameter  calDispType=Number  calEnum={'False', 'True'}  calGain=1.0  calOffset=0.0  calMax=inf  calMin=-inf  calFormat='-1'  calUnit=''  calHelp=''  calAccess=1  calFunction=raptor_xcp_function(gcb)  calVisible=on
      settings: SourceProductName=Raptor
  raptor_measurement1 : Raptor_lib/Data Storage/raptor_measurement  paramName='T14'  nameSource=Parameter  calDispType=Number  calEnum={'False', 'True'}  calGain=1.0  calOffset=0.0  calMax=inf  calMin=-inf  calFormat='-1'  calUnit=''  calHelp=''  calAccess=1  calFunction=raptor_xcp_function(gcb)  calVisible=on
      settings: SourceProductName=Raptor
  raptor_measurement2 : Raptor_lib/Data Storage/raptor_measurement  paramName='T15'  nameSource=Parameter  calDispType=Number  calEnum={'False', 'True'}  calGain=1.0  calOffset=0.0  calMax=inf  calMin=-inf  calFormat='-1'  calUnit=''  calHelp=''  calAccess=1  calFunction=raptor_xcp_function(gcb)  calVisible=on
      settings: SourceProductName=Raptor
  raptor_measurement3 : Raptor_lib/Data Storage/raptor_measurement  paramName='T16'  nameSource=Parameter  calDispType=Number  calEnum={'False', 'True'}  calGain=1.0  calOffset=0.0  calMax=inf  calMin=-inf  calFormat='-1'  calUnit=''  calHelp=''  calAccess=1  calFunction=raptor_xcp_function(gcb)  calVisible=on
      settings: SourceProductName=Raptor
  wires:
  Demux/8 -> Convert_Byte2Data3/1(HighByte)
  Demux/7 -> Convert_Byte2Data3/2(LowByte)
  Demux/6 -> Convert_Byte2Data2/1(HighByte)
  Demux/5 -> Convert_Byte2Data2/2(LowByte)
  Demux/1 -> Convert_Byte2Data/2(LowByte)
  Demux/2 -> Convert_Byte2Data/1(HighByte)
  Demux/3 -> Convert_Byte2Data1/2(LowByte)
  Demux/4 -> Convert_Byte2Data1/1(HighByte)
  Offset/1 -> Convert_Byte2Data3/3(Offset), Convert_Byte2Data2/3(Offset), Convert_Byte2Data1/3(Offset), Convert_Byte2Data/3(Offset)
  Factor/1 -> Convert_Byte2Data3/4(Factor), Convert_Byte2Data2/4(Factor), Convert_Byte2Data1/4(Factor), Convert_Byte2Data/4(Factor)
  Convert_Byte2Data2/1(Data) -> raptor_measurement2/1
  Convert_Byte2Data3/1(Data) -> raptor_measurement3/1
  raptor_can_rxraw/5 -> Demux/1
  Convert_Byte2Data/1(Data) -> raptor_measurement/1
  Convert_Byte2Data1/1(Data) -> raptor_measurement1/1

== system EPT/Foreground_TimeBase_5ms/CAN/CAN3_exec/20CH_TCS/CH17_CH20_Rx1 ==
  Factor : Inport
  Offset : Inport  Port=2
  Trigger : TriggerPort  VariantControl=Variant  PortDimensions=1
  Convert_Byte2Data : Subsystem
  Convert_Byte2Data1 : Subsystem
  Convert_Byte2Data2 : Subsystem
  Convert_Byte2Data3 : Subsystem
  Demux : Demux  Outputs=8
  raptor_can_rxraw : Raptor_lib/CAN/raptor_can_rxraw  canBus='CAN3'  extendedId=1  showAge=1  id=hex2dec('18FE9FEB')  idMask=hex2dec('1FFFFFFF')  mailbox=''  queueSize=1
      settings: SourceProductName=Raptor
  raptor_measurement : Raptor_lib/Data Storage/raptor_measurement  paramName='T17'  nameSource=Parameter  calDispType=Number  calEnum={'False', 'True'}  calGain=1.0  calOffset=0.0  calMax=inf  calMin=-inf  calFormat='-1'  calUnit=''  calHelp=''  calAccess=1  calFunction=raptor_xcp_function(gcb)  calVisible=on
      settings: SourceProductName=Raptor
  raptor_measurement1 : Raptor_lib/Data Storage/raptor_measurement  paramName='T18'  nameSource=Parameter  calDispType=Number  calEnum={'False', 'True'}  calGain=1.0  calOffset=0.0  calMax=inf  calMin=-inf  calFormat='-1'  calUnit=''  calHelp=''  calAccess=1  calFunction=raptor_xcp_function(gcb)  calVisible=on
      settings: SourceProductName=Raptor
  raptor_measurement2 : Raptor_lib/Data Storage/raptor_measurement  paramName='T19'  nameSource=Parameter  calDispType=Number  calEnum={'False', 'True'}  calGain=1.0  calOffset=0.0  calMax=inf  calMin=-inf  calFormat='-1'  calUnit=''  calHelp=''  calAccess=1  calFunction=raptor_xcp_function(gcb)  calVisible=on
      settings: SourceProductName=Raptor
  raptor_measurement3 : Raptor_lib/Data Storage/raptor_measurement  paramName='T20'  nameSource=Parameter  calDispType=Number  calEnum={'False', 'True'}  calGain=1.0  calOffset=0.0  calMax=inf  calMin=-inf  calFormat='-1'  calUnit=''  calHelp=''  calAccess=1  calFunction=raptor_xcp_function(gcb)  calVisible=on
      settings: SourceProductName=Raptor
  wires:
  Convert_Byte2Data1/1(Data) -> raptor_measurement1/1
  Convert_Byte2Data/1(Data) -> raptor_measurement/1
  raptor_can_rxraw/5 -> Demux/1
  Convert_Byte2Data3/1(Data) -> raptor_measurement3/1
  Convert_Byte2Data2/1(Data) -> raptor_measurement2/1
  Factor/1 -> Convert_Byte2Data3/4(Factor), Convert_Byte2Data2/4(Factor), Convert_Byte2Data1/4(Factor), Convert_Byte2Data/4(Factor)
  Offset/1 -> Convert_Byte2Data3/3(Offset), Convert_Byte2Data2/3(Offset), Convert_Byte2Data1/3(Offset), Convert_Byte2Data/3(Offset)
  Demux/4 -> Convert_Byte2Data1/1(HighByte)
  Demux/3 -> Convert_Byte2Data1/2(LowByte)
  Demux/2 -> Convert_Byte2Data/1(HighByte)
  Demux/1 -> Convert_Byte2Data/2(LowByte)
  Demux/5 -> Convert_Byte2Data2/2(LowByte)
  Demux/6 -> Convert_Byte2Data2/1(HighByte)
  Demux/7 -> Convert_Byte2Data3/2(LowByte)
  Demux/8 -> Convert_Byte2Data3/1(HighByte)

== system EPT/Foreground_TimeBase_5ms/CAN/CAN3_exec/20CH_TCS/CH1_CH4_Rx ==
  Factor : Inport
  Offset : Inport  Port=2
  Trigger : TriggerPort  VariantControl=Variant  PortDimensions=1
  Convert_Byte2Data : Subsystem
  Convert_Byte2Data1 : Subsystem
  Convert_Byte2Data2 : Subsystem
  Convert_Byte2Data3 : Subsystem
  Demux : Demux  Outputs=8
  raptor_can_rxraw : Raptor_lib/CAN/raptor_can_rxraw  canBus='CAN3'  extendedId=1  showAge=1  id=hex2dec('18FEA3EB')  idMask=hex2dec('1FFFFFFF')  mailbox=''  queueSize=1
      settings: SourceProductName=Raptor
  raptor_measurement : Raptor_lib/Data Storage/raptor_measurement  paramName='T01'  nameSource=Parameter  calDispType=Number  calEnum={'False', 'True'}  calGain=1.0  calOffset=0.0  calMax=inf  calMin=-inf  calFormat='-1'  calUnit=''  calHelp=''  calAccess=1  calFunction=raptor_xcp_function(gcb)  calVisible=on
      settings: SourceProductName=Raptor
  raptor_measurement1 : Raptor_lib/Data Storage/raptor_measurement  paramName='T02'  nameSource=Parameter  calDispType=Number  calEnum={'False', 'True'}  calGain=1.0  calOffset=0.0  calMax=inf  calMin=-inf  calFormat='-1'  calUnit=''  calHelp=''  calAccess=1  calFunction=raptor_xcp_function(gcb)  calVisible=on
      settings: SourceProductName=Raptor
  raptor_measurement2 : Raptor_lib/Data Storage/raptor_measurement  paramName='T03'  nameSource=Parameter  calDispType=Number  calEnum={'False', 'True'}  calGain=1.0  calOffset=0.0  calMax=inf  calMin=-inf  calFormat='-1'  calUnit=''  calHelp=''  calAccess=1  calFunction=raptor_xcp_function(gcb)  calVisible=on
      settings: SourceProductName=Raptor
  raptor_measurement3 : Raptor_lib/Data Storage/raptor_measurement  paramName='T04'  nameSource=Parameter  calDispType=Number  calEnum={'False', 'True'}  calGain=1.0  calOffset=0.0  calMax=inf  calMin=-inf  calFormat='-1'  calUnit=''  calHelp=''  calAccess=1  calFunction=raptor_xcp_function(gcb)  calVisible=on
      settings: SourceProductName=Raptor
  raptor_measurement4 : Raptor_lib/Data Storage/raptor_measurement  paramName='Age_20CH_TCS'  nameSource=Parameter  calDispType=Number  calEnum={'False', 'True'}  calGain=1.0  calOffset=0.0  calMax=inf  calMin=-inf  calFormat='-1'  calUnit=''  calHelp=''  calAccess=1  calFunction=raptor_xcp_function(gcb)  calVisible=on
      settings: SourceProductName=Raptor
  wires:
  Convert_Byte2Data1/1(Data) -> raptor_measurement1/1
  Convert_Byte2Data/1(Data) -> raptor_measurement/1
  raptor_can_rxraw/5 -> Demux/1
  Convert_Byte2Data3/1(Data) -> raptor_measurement3/1
  Convert_Byte2Data2/1(Data) -> raptor_measurement2/1
  Factor/1 -> Convert_Byte2Data3/4(Factor), Convert_Byte2Data2/4(Factor), Convert_Byte2Data1/4(Factor), Convert_Byte2Data/4(Factor)
  Offset/1 -> Convert_Byte2Data3/3(Offset), Convert_Byte2Data2/3(Offset), Convert_Byte2Data1/3(Offset), Convert_Byte2Data/3(Offset)
  Demux/4 -> Convert_Byte2Data1/1(HighByte)
  Demux/3 -> Convert_Byte2Data1/2(LowByte)
  Demux/2 -> Convert_Byte2Data/1(HighByte)
  Demux/1 -> Convert_Byte2Data/2(LowByte)
  Demux/5 -> Convert_Byte2Data2/2(LowByte)
  Demux/6 -> Convert_Byte2Data2/1(HighByte)
  Demux/7 -> Convert_Byte2Data3/2(LowByte)
  Demux/8 -> Convert_Byte2Data3/1(HighByte)
  raptor_can_rxraw/1 -> raptor_measurement4/1

== system EPT/Foreground_TimeBase_5ms/CAN/CAN3_exec/20CH_TCS/CH5_CH8_Rx ==
  Factor : Inport
  Offset : Inport  Port=2
  Trigger : TriggerPort  VariantControl=Variant  PortDimensions=1
  Convert_Byte2Data : Subsystem
  Convert_Byte2Data1 : Subsystem
  Convert_Byte2Data2 : Subsystem
  Convert_Byte2Data3 : Subsystem
  Demux : Demux  Outputs=8
  raptor_can_rxraw : Raptor_lib/CAN/raptor_can_rxraw  canBus='CAN3'  extendedId=1  showAge=1  id=hex2dec('18FEA2EB')  idMask=hex2dec('1FFFFFFF')  mailbox=''  queueSize=1
      settings: SourceProductName=Raptor
  raptor_measurement : Raptor_lib/Data Storage/raptor_measurement  paramName='T05'  nameSource=Parameter  calDispType=Number  calEnum={'False', 'True'}  calGain=1.0  calOffset=0.0  calMax=inf  calMin=-inf  calFormat='-1'  calUnit=''  calHelp=''  calAccess=1  calFunction=raptor_xcp_function(gcb)  calVisible=on
      settings: SourceProductName=Raptor
  raptor_measurement1 : Raptor_lib/Data Storage/raptor_measurement  paramName='T06'  nameSource=Parameter  calDispType=Number  calEnum={'False', 'True'}  calGain=1.0  calOffset=0.0  calMax=inf  calMin=-inf  calFormat='-1'  calUnit=''  calHelp=''  calAccess=1  calFunction=raptor_xcp_function(gcb)  calVisible=on
      settings: SourceProductName=Raptor
  raptor_measurement2 : Raptor_lib/Data Storage/raptor_measurement  paramName='T07'  nameSource=Parameter  calDispType=Number  calEnum={'False', 'True'}  calGain=1.0  calOffset=0.0  calMax=inf  calMin=-inf  calFormat='-1'  calUnit=''  calHelp=''  calAccess=1  calFunction=raptor_xcp_function(gcb)  calVisible=on
      settings: SourceProductName=Raptor
  raptor_measurement3 : Raptor_lib/Data Storage/raptor_measurement  paramName='T08'  nameSource=Parameter  calDispType=Number  calEnum={'False', 'True'}  calGain=1.0  calOffset=0.0  calMax=inf  calMin=-inf  calFormat='-1'  calUnit=''  calHelp=''  calAccess=1  calFunction=raptor_xcp_function(gcb)  calVisible=on
      settings: SourceProductName=Raptor
  wires:
  Demux/8 -> Convert_Byte2Data3/1(HighByte)
  Demux/7 -> Convert_Byte2Data3/2(LowByte)
  Demux/6 -> Convert_Byte2Data2/1(HighByte)
  Demux/5 -> Convert_Byte2Data2/2(LowByte)
  Demux/1 -> Convert_Byte2Data/2(LowByte)
  Demux/2 -> Convert_Byte2Data/1(HighByte)
  Demux/3 -> Convert_Byte2Data1/2(LowByte)
  Demux/4 -> Convert_Byte2Data1/1(HighByte)
  Offset/1 -> Convert_Byte2Data3/3(Offset), Convert_Byte2Data2/3(Offset), Convert_Byte2Data1/3(Offset), Convert_Byte2Data/3(Offset)
  Factor/1 -> Convert_Byte2Data3/4(Factor), Convert_Byte2Data2/4(Factor), Convert_Byte2Data1/4(Factor), Convert_Byte2Data/4(Factor)
  Convert_Byte2Data2/1(Data) -> raptor_measurement2/1
  Convert_Byte2Data3/1(Data) -> raptor_measurement3/1
  raptor_can_rxraw/5 -> Demux/1
  Convert_Byte2Data/1(Data) -> raptor_measurement/1
  Convert_Byte2Data1/1(Data) -> raptor_measurement1/1

== system EPT/Foreground_TimeBase_5ms/CAN/CAN3_exec/20CH_TCS/CH9_CH12_Rx ==
  Factor : Inport
  Offset : Inport  Port=2
  Trigger : TriggerPort  VariantControl=Variant  PortDimensions=1
  Convert_Byte2Data : Subsystem
  Convert_Byte2Data1 : Subsystem
  Convert_Byte2Data2 : Subsystem
  Convert_Byte2Data3 : Subsystem
  Demux : Demux  Outputs=8
  raptor_can_rxraw : Raptor_lib/CAN/raptor_can_rxraw  canBus='CAN3'  extendedId=1  showAge=1  id=hex2dec('18FEA1EB')  idMask=hex2dec('1FFFFFFF')  mailbox=''  queueSize=1
      settings: SourceProductName=Raptor
  raptor_measurement : Raptor_lib/Data Storage/raptor_measurement  paramName='T09'  nameSource=Parameter  calDispType=Number  calEnum={'False', 'True'}  calGain=1.0  calOffset=0.0  calMax=inf  calMin=-inf  calFormat='-1'  calUnit=''  calHelp=''  calAccess=1  calFunction=raptor_xcp_function(gcb)  calVisible=on
      settings: SourceProductName=Raptor
  raptor_measurement1 : Raptor_lib/Data Storage/raptor_measurement  paramName='T10'  nameSource=Parameter  calDispType=Number  calEnum={'False', 'True'}  calGain=1.0  calOffset=0.0  calMax=inf  calMin=-inf  calFormat='-1'  calUnit=''  calHelp=''  calAccess=1  calFunction=raptor_xcp_function(gcb)  calVisible=on
      settings: SourceProductName=Raptor
  raptor_measurement2 : Raptor_lib/Data Storage/raptor_measurement  paramName='T11'  nameSource=Parameter  calDispType=Number  calEnum={'False', 'True'}  calGain=1.0  calOffset=0.0  calMax=inf  calMin=-inf  calFormat='-1'  calUnit=''  calHelp=''  calAccess=1  calFunction=raptor_xcp_function(gcb)  calVisible=on
      settings: SourceProductName=Raptor
  raptor_measurement3 : Raptor_lib/Data Storage/raptor_measurement  paramName='T12'  nameSource=Parameter  calDispType=Number  calEnum={'False', 'True'}  calGain=1.0  calOffset=0.0  calMax=inf  calMin=-inf  calFormat='-1'  calUnit=''  calHelp=''  calAccess=1  calFunction=raptor_xcp_function(gcb)  calVisible=on
      settings: SourceProductName=Raptor
  wires:
  Convert_Byte2Data1/1(Data) -> raptor_measurement1/1
  Convert_Byte2Data/1(Data) -> raptor_measurement/1
  raptor_can_rxraw/5 -> Demux/1
  Convert_Byte2Data3/1(Data) -> raptor_measurement3/1
  Convert_Byte2Data2/1(Data) -> raptor_measurement2/1
  Factor/1 -> Convert_Byte2Data3/4(Factor), Convert_Byte2Data2/4(Factor), Convert_Byte2Data1/4(Factor), Convert_Byte2Data/4(Factor)
  Offset/1 -> Convert_Byte2Data3/3(Offset), Convert_Byte2Data2/3(Offset), Convert_Byte2Data1/3(Offset), Convert_Byte2Data/3(Offset)
  Demux/4 -> Convert_Byte2Data1/1(HighByte)
  Demux/3 -> Convert_Byte2Data1/2(LowByte)
  Demux/2 -> Convert_Byte2Data/1(HighByte)
  Demux/1 -> Convert_Byte2Data/2(LowByte)
  Demux/5 -> Convert_Byte2Data2/2(LowByte)
  Demux/6 -> Convert_Byte2Data2/1(HighByte)
  Demux/7 -> Convert_Byte2Data3/2(LowByte)
  Demux/8 -> Convert_Byte2Data3/1(HighByte)

== system EPT/Foreground_TimeBase_5ms/CAN/CAN3_exec/20CH_TCS/CountTrigger ==
  Counter : Inport
  Constant1 : Constant  Value=0
  Constant3 : Constant
  CycleTrigger : Subsystem
  Switch : Switch  Threshold=1
  Unit Delay : UnitDelay  SampleTime=-1  HasFrameUpgradeWarning=on
  Tirgger : Outport  VectorParamsAs1DForOutWhenUnconnected=off
  wires:
  Unit Delay/1 -> Switch/2
  CycleTrigger/1(Trigger) -> Unit Delay/1, Tirgger/1
  Counter/1 -> CycleTrigger/2(In2)
  Constant1/1 -> Switch/1
  Constant3/1 -> Switch/3
  Switch/1 -> CycleTrigger/1(In1)

== system EPT/Foreground_TimeBase_5ms/CAN/CAN3_exec/DCDC/CountTrigger ==
  Counter : Inport
  Constant1 : Constant  Value=0
  Constant3 : Constant
  CycleTrigger : Subsystem
  Switch : Switch  Threshold=1
  Unit Delay1 : UnitDelay  SampleTime=-1  HasFrameUpgradeWarning=on
  Unit Delay2 : UnitDelay  SampleTime=-1  HasFrameUpgradeWarning=on
  Tirgger : Outport  VectorParamsAs1DForOutWhenUnconnected=off
  wires:
  Unit Delay2/1 -> Tirgger/1
  Unit Delay1/1 -> CycleTrigger/1(In1)
  CycleTrigger/1(Trigger) -> Unit Delay2/1, Switch/2
  Counter/1 -> CycleTrigger/2(In2)
  Constant1/1 -> Switch/1
  Constant3/1 -> Switch/3
  Switch/1 -> Unit Delay1/1
